simulink model "PVPAPERFULL"  (R2021b)
settings: Solver=VariableStepAuto  StartTime=0.0  StopTime=30.0  FixedStep=0.01  RelTol=1e-3
libraries: simulink x2, spsControlledCurrentSourceLib x1, spsControlledVoltageSourceLib x1, spsCurrentMeasurementLib x1, spsDiodeLib x1, spsVoltageMeasurementLib x1, spspowerguiLib x1
settings Model: Creator=shiuanlee  LastModifiedBy=Shiuan

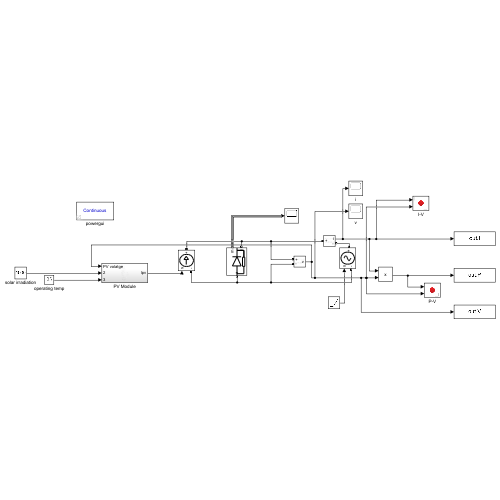
[thumbnail: Simulink's stored preview of the top-level diagram]
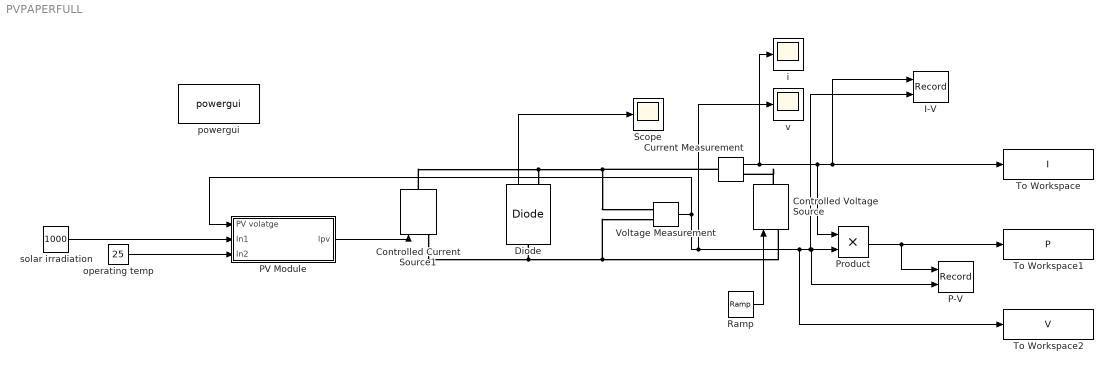
== system PVPAPERFULL ==
  Controlled Current Source1 : spsControlledCurrentSourceLib/Controlled Current Source  Initialize=on  Source_Type=AC  Amplitude=0  Phase=0  Frequency=0  Measurements=None
  Controlled Voltage Source : spsControlledVoltageSourceLib/Controlled Voltage Source  Initialize=on  Source_Type=AC  Amplitude=0  Phase=0  Frequency=0  Measurements=None
  Current Measurement : spsCurrentMeasurementLib/Current Measurement  PhasorSimulation=off  OutputType=Complex  PSBequivalent=0
  Diode : spsDiodeLib/Diode  Ron=0.001  Lon=0  Vf=0.8  IC=0  UseSnubber=0  Rs=500  Cs=250e-9  Measurements=on
  I-V : Record  FileSettingsInternal="{\"entries\":[{\"content\":{\"excelSettings\":{\"content\":{},\"type\":\"Streamout.ExcelSettings\"}},\"type\":\"Streamout.FileSettingStorage\",\"uuid\":\"36aaff03-e2d8-4f23-a0c3-637c8ac80c8f\"}],\"packageUris\":[\"http://schema.mathworks.com/mf0/streamout_blocks/R2020a\"],\"version\":\"1.0\"}"  Layout=[1 1]  SignalsInternal="{\"entries\":[{\"content\":{\"signals\":[{\"content\":{\"blockPath\":[\"PVPAPERFULL/I-V\"],\"channel\":[],\"dimensions\":[1],\"domain\":\"PVPAPERFULL/I-V\",\"lineColor\":\"#139fff\",\"plots\":[],\"port\":1,\"sid\":[\"\"],\"signalID\":2561,\"signalName\":\"Current Measurement\"},\"type\":\"RecordBlkView.Signal\",\"uuid\":\"db08aa17-c25b-43ab-bd0f-8571df5a55c5\"},{\"content\":{\"blockPath\":[\"PVPAPERFULL/I-V\"],\"channel\":[],\"dimensions\":[1],\"domain\":\"PVPAPERFULL/I-V\",\"lineColor\":\"#ff6929\",\"plots\":[],\"port\":2,\"sid\":[\"\"],\"signalID\":2565,\"signalName\":\"Voltage Measurement\"},\"type\":\"RecordBlkView.Signal\",\"uuid\":\"16e919e3-9877-4a22-964a-cc0445c3d14e\"}]},\"type\":\"RecordBlkView.InputSignals\",\"uuid\":\"2386edbf-e72d-401e-9176-175722332550\"}],\"packageUris\":[\"http://schema.mathworks.com/mf0/streamout_blocks/R2020a\"],\"version\":\"1.0\"}"  VisualizationBindings="{\"xyplotplugin\":{\"info\":[{\"series\":[],\"subplotID\":1}]}}"  CompatibilityTag=XY
  P-V : Record  FileSettingsInternal="{\"entries\":[{\"content\":{\"excelSettings\":{\"content\":{},\"type\":\"Streamout.ExcelSettings\"}},\"type\":\"Streamout.FileSettingStorage\",\"uuid\":\"6adaefe9-4cd2-429f-9127-09dd1fe31cef\"}],\"packageUris\":[\"http://schema.mathworks.com/mf0/streamout_blocks/R2020a\"],\"version\":\"1.0\"}"  Layout=[1 1]  SignalsInternal="{\"entries\":[{\"content\":{\"signals\":[{\"content\":{\"blockPath\":[\"PVPAPERFULL/P-V\"],\"channel\":[],\"dimensions\":[1],\"domain\":\"PVPAPERFULL/P-V\",\"lineColor\":\"#b746ff\",\"plots\":[],\"port\":1,\"sid\":[\"\"],\"signalID\":2569,\"signalName\":\"Product\"},\"type\":\"RecordBlkView.Signal\",\"uuid\":\"2bab4d67-adbc-4489-bddd-a9c0aabdc29e\"},{\"content\":{\"blockPath\":[\"PVPAPERFULL/P-V\"],\"channel\":[],\"dimensions\":[1],\"domain\":\"PVPAPERFULL/P-V\",\"lineColor\":\"#64d413\",\"plots\":[],\"port\":2,\"sid\":[\"\"],\"signalID\":2573,\"signalName\":\"Voltage Measurement\"},\"type\":\"RecordBlkView.Signal\",\"uuid\":\"ece211cf-a2a6-4dbd-807b-14eb8ce103a1\"}]},\"type\":\"RecordBlkView.InputSignals\",\"uuid\":\"0634f269-aaca-4857-9a94-01b50dbf8e93\"}],\"packageUris\":[\"http://schema.mathworks.com/mf0/streamout_blocks/R2020a\"],\"version\":\"1.0\"}"  VisualizationBindings="{\"xyplotplugin\":{\"info\":[{\"series\":[],\"subplotID\":1}]}}"  CompatibilityTag=XY
  PV Module : Subsystem
  Product : Product
  Ramp : simulink/Sources/Ramp  slope=1  start=0  InitialOutput=0
  Scope : Scope
  To Workspace : ToWorkspace  VariableName=I  SampleTime=-1
      settings: Save2DSignal=2-D array (concatenate along first dimension)
  To Workspace1 : ToWorkspace  VariableName=P  SampleTime=-1
      settings: Save2DSignal=2-D array (concatenate along first dimension)
  To Workspace2 : ToWorkspace  VariableName=V  SampleTime=-1
      settings: Save2DSignal=2-D array (concatenate along first dimension)
  Voltage Measurement : spsVoltageMeasurementLib/Voltage Measurement  PhasorSimulation=off  OutputType=Complex  PSBequivalent=0
  i : Scope
  operating temp : Constant  Value=25
  powergui : spspowerguiLib/powergui  Priority=1  SimulationMode=Continuous  SampleTime=50e-6  frequency=60  Iterations=50  frequencyindice=0  Pbase=100e6  ErrMax=1e-4  UnitsV=kV  UnitsW=MW  buscounter=0  FunctionMessages=off  echomessages=off  EnableUseOfTLC=off  CurrentSourceSwitches=off  DisableSnubberDevices=off  DisableRonSwitches=off  DisableVfSwitches=off  DisplayEquations=off  AutomaticDiscreteSolvers=off  SolverType=Tustin/Backward Euler (TBE)  Interpol=off  ExternalGateDelay=off  methode=off  Ts=100  x0status=blocks  SPID=on  SwTol=0  HookPort=off  NonlinearTolerance=1e-4  nMaxIteration=100  ContinueOnMaxIteration=off  RestoreLinks=warning  ResistiveCurrentMeasurement=off  Frange=[0:2:500]  Ylog=off  Xlog=on  ShowGrid=off  save=off  variable=ZData  structure=0  ZoomFFT=off  StartTime=0.0  cycles=1  DisplayStyle=1  fundamental=60  FreqAxis=off  MaxFrequency=1000  frequencyindicesteady=1  RmsSteady=1  display=off
  solar irradiation : Constant  Value=1000
  v : Scope
  wires:
  solar irradiation/1 -> PV Module/2(In1)
  operating temp/1 -> PV Module/3(In2)
  PV Module/1(lpv) -> Controlled Current Source1/1
  Diode/1 -> Scope/1
  Voltage Measurement/1 -> PV Module/1(PV volatge), I-V/2, P-V/2, Product/2, To Workspace2/1, v/1
  Ramp/1 -> Controlled Voltage Source/1
  Product/1 -> P-V/1, To Workspace1/1
  Current Measurement/1 -> i/1, Product/1, I-V/1, To Workspace/1
  connections:
  Controlled Current Source1/RConn1 -- Current Measurement/LConn1 -- Voltage Measurement/LConn1 -- Diode/RConn1
  Controlled Current Source1/LConn1 -- Voltage Measurement/LConn2 -- Controlled Voltage Source/LConn1 -- Diode/LConn1
  Controlled Voltage Source/RConn1 -- Current Measurement/RConn1

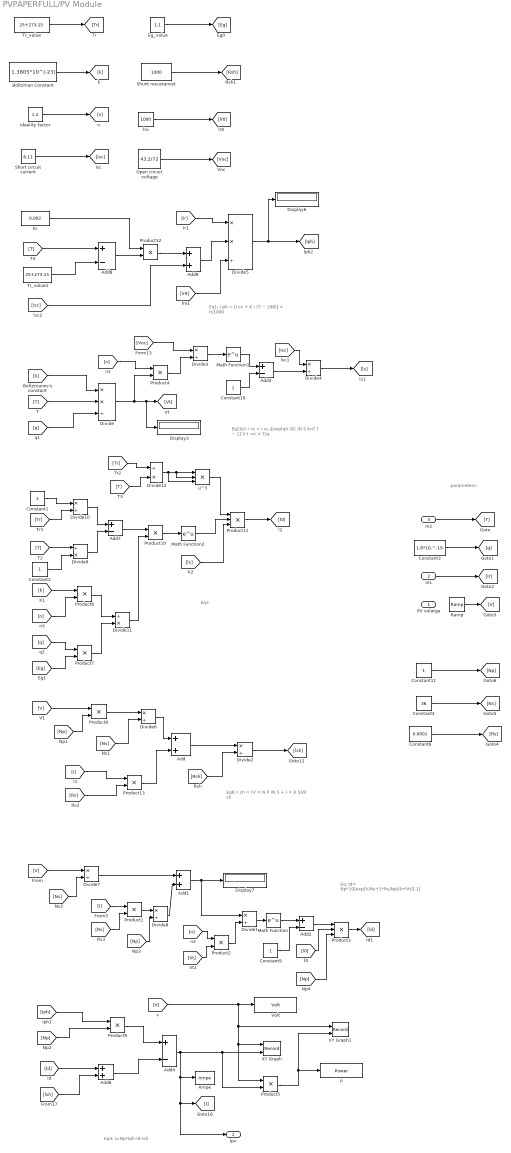
== system PVPAPERFULL/PV Module ==
  note: Eq4:
      | I=Np*Iph-Id-Ish
  note: Eq6:
      | I sh = (V × N P /N S + I × R S)/R sh
  note: Eq1:
      | I ph = [I sc + K i (T − 298)] × Ir/1000
  note: Eq:
      | Id= Np*10[exp[V/Ns+1*Rs/Np)/(n*Vt)]-1]
  note: Eq2&5:
      | I rs = I sc /[exp(qV OC /N S knT ) − 1]
      | V t =k × T/q
  note: parameters:
  note: Eq3
  PV volatge : Inport
  In1 : Inport  Port=2
  In2 : Inport  Port=3
  Add{,1,6,9} (4 alike) : Sum
  Add{2..4,7..8} (5 alike) : Sum  Inputs=+-
  Ampe : ToWorkspace  VariableName=Ampe  SaveFormat=Timeseries  SampleTime=-1
  Boltzman Constant : Constant  Value=1.3805*10^(-23)
  Constant{1..2,9..11} (5 alike) : Constant
  Constant3 : Constant  Value=1.6*10.^-19
  Constant4 : Constant  Value=36
  Constant6 : Constant  Value=0.0001
  Display3 : Display
  Display6 : Display
  Display7 : Display
  Divide : Product  Inputs=**/
  Divide{1..4,6..8,10} (8 alike) : Product  Inputs=*/
  Divide11 : Product  Inputs=/*
  Divide12 : Product  Inputs=/*
  Divide5 : Product  Inputs=**/
  Divide9 : Product  Inputs=/*
  Eg_value : Constant  Value=1.1
  Ideality factor : Constant  Value=1.2
  Ki : Constant  Value=0.002
  Math Function : Math  SaturateOnIntegerOverflow=on
  Math Function1 : Math  SaturateOnIntegerOverflow=on
  Math Function2 : Math  SaturateOnIntegerOverflow=on
  Open circuit voltage : Constant  Value=43.2/72
  P : ToWorkspace  VariableName=Power  SaveFormat=Timeseries  SampleTime=-1
  Product{1..2,4..10,12..13} (11 alike) : Product
  Product11 : Product  Inputs=3
  Product3 : Product  Inputs=3
  Ramp : simulink/Sources/Ramp  slope=1  start=0  InitialOutput=0
  Short circuit current : Constant  Value=6.11
  Shunt resustancet : Constant  Value=1000
  Tr_value : Constant  Value=25+273.15
  Tr_value1 : Constant  Value=25+273.15
  Volt : ToWorkspace  VariableName=Volt  SaveFormat=Timeseries  SampleTime=-1
  XY Graph : Record  FileSettingsInternal="{\"entries\":[{\"content\":{\"excelSettings\":{\"content\":{},\"type\":\"Streamout.ExcelSettings\"}},\"type\":\"Streamout.FileSettingStorage\",\"uuid\":\"ab1ddb20-419f-491b-9c58-684249219fa2\"}],\"packageUris\":[\"http://schema.mathworks.com/mf0/streamout_blocks/R2020a\"],\"version\":\"1.0\"}"  Layout=[1 1]  SignalsInternal="{\"entries\":[{\"content\":{\"signals\":[{\"content\":{\"blockPath\":[\"PVPAPERFULL/PV Module/XY Graph\"],\"channel\":[],\"dimensions\":[1],\"domain\":\"PVPAPERFULL/PV Module/XY Graph\",\"lineColor\":\"#ff13a6\",\"plots\":[],\"port\":1,\"sid\":[\"\"],\"signalID\":2577,\"signalName\":\"v\"},\"type\":\"RecordBlkView.Signal\",\"uuid\":\"b3b8c47f-d49e-40f3-9268-4f0746602f4a\"},{\"content\":{\"blockPath\":[\"PVPAPERFULL/PV Module/XY Graph\"],\"channel\":[],\"dimensions\":[1],\"domain\":\"PVPAPERFULL/PV Module/XY Graph\",\"lineColor\":\"#fe330a\",\"plots\":[],\"port\":2,\"sid\":[\"\"],\"signalID\":2581,\"signalName\":\"Add4\"},\"type\":\"RecordBlkView.Signal\",\"uuid\":\"6a1236be-1971-4489-abe7-72c75e1e56dd\"}]},\"type\":\"RecordBlkView.InputSignals\",\"uuid\":\"4581ca48-da48-410f-b8a3-f7acb8399d5c\"}],\"packageUris\":[\"http://schema.mathworks.com/mf0/streamout_blocks/R2020a\"],\"version\":\"1.0\"}"  CompatibilityTag=XY
  XY Graph1 : Record  FileSettingsInternal="{\"entries\":[{\"content\":{\"excelSettings\":{\"content\":{},\"type\":\"Streamout.ExcelSettings\"}},\"type\":\"Streamout.FileSettingStorage\",\"uuid\":\"4447556a-2442-499e-ba43-95e3cd0e45cb\"}],\"packageUris\":[\"http://schema.mathworks.com/mf0/streamout_blocks/R2020a\"],\"version\":\"1.0\"}"  Layout=[1 1]  SignalsInternal="{\"entries\":[{\"content\":{\"signals\":[{\"content\":{\"blockPath\":[\"PVPAPERFULL/PV Module/XY Graph1\"],\"channel\":[],\"dimensions\":[1],\"domain\":\"PVPAPERFULL/PV Module/XY Graph1\",\"lineColor\":\"#22b573\",\"plots\":[],\"port\":1,\"sid\":[\"\"],\"signalID\":2585,\"signalName\":\"v\"},\"type\":\"RecordBlkView.Signal\",\"uuid\":\"bc056c73-eab7-4f39-8a85-5b50627b3442\"},{\"content\":{\"blockPath\":[\"PVPAPERFULL/PV Module/XY Graph1\"],\"channel\":[],\"dimensions\":[1],\"domain\":\"PVPAPERFULL/PV Module/XY Graph1\",\"lineColor\":\"#0072bd\",\"plots\":[],\"port\":2,\"sid\":[\"\"],\"signalID\":2589,\"signalName\":\"Product5\"},\"type\":\"RecordBlkView.Signal\",\"uuid\":\"cc3d43ba-43ff-43cb-8563-964e4b65ad12\"}]},\"type\":\"RecordBlkView.InputSignals\",\"uuid\":\"8793bc40-c625-4f15-adda-cfc5e14292cf\"}],\"packageUris\":[\"http://schema.mathworks.com/mf0/streamout_blocks/R2020a\"],\"version\":\"1.0\"}"  VisualizationBindings="{\"xyplotplugin\":{\"info\":[{\"series\":[],\"subplotID\":1}]}}"  CompatibilityTag=XY
  lro : Constant  Value=1000
  u^3 : Product  Inputs=3
  lpv : Outport
  wires:
  [Np] -> Product9/2
  [ld] -> Add6/1
  Divide1/1 -> Math Function/1
  Product3/1 -> [ld]
  Constant9/1 -> Add2/2
  Boltzman Constant/1 -> [k]
  Math Function1/1 -> Add3/1
  [Tr] -> Divide12/1
  Divide9/1 -> Add7/2
  Product5/1 -> XY Graph1/2, P/1
  [Np] -> Divide8/2
  Tr_value1/1 -> Add8/2
  Constant11/1 -> [Np]
  [lsh] -> Add6/2
  [V] -> Volt/1, XY Graph1/1, Product5/1, XY Graph/1
  Tr_value/1 -> [Tr]
  Ki/1 -> Product12/1
  Product12/1 -> Add9/1
  [n] -> Product6/2
  [Vt] -> Product2/2
  Product7/1 -> Divide11/2
  Math Function2/1 -> Product11/2
  Constant3/1 -> [q]
  Constant4/1 -> [Ns]
  Product10/1 -> Math Function2/1
  [Ns] -> Divide7/2
  Math Function/1 -> Add2/1
  [lr0] -> Divide5/3
  [Np] -> Product3/3
  [Iph] -> Product9/1
  [ls] -> Product11/3
  Constant6/1 -> [Rs]
  Constant2/1 -> Divide9/2
  Divide/1 -> Display3/1, [Vt], Product4/2
  Constant10/1 -> Add3/2
  Divide2/1 -> [lsh]
  Add2/1 -> Product3/1
  [T] -> Divide12/2
  Product2/1 -> Divide1/2
  [I] -> Product1/1
  Product1/1 -> Divide8/1
  [l0] -> Product3/2
  Divide8/1 -> Add1/2
  [n] -> Product2/1
  Product13/1 -> Add/2
  Add1/1 -> Divide1/1, Display7/1
  Open circuit voltage/1 -> [Voc]
  [V] -> Divide7/1
  [Ns] -> Divide6/2
  [Rs] -> Product1/2
  [k] -> Product6/1
  [Isc] -> Add9/2
  Divide3/1 -> Math Function1/1
  [T] -> Add8/1
  Ideality factor/1 -> [n]
  Product8/1 -> Divide6/1
  [Tr] -> Divide10/2
  Add7/1 -> Product10/1
  [V] -> Product8/1
  [q] -> Product7/1
  Divide11/1 -> Product10/2
  Divide10/1 -> Add7/1
  [Np] -> Product8/2
  [T] -> Divide9/1
  u^3/1 -> Product11/1
  Product6/1 -> Divide11/1
  Constant1/1 -> Divide10/1
  Product11/1 -> [l0]
  [Eg] -> Product7/2
  [Isc] -> Divide4/1
  [k] -> Divide/1
  Divide6/1 -> Add/1
  Add8/1 -> Product12/2
  [Rs] -> Product13/2
  Product4/1 -> Divide3/2
  lro/1 -> [lr0]
  [Rsh] -> Divide2/2
  Divide12/1 -> u^3/3, u^3/2, u^3/1
  [n] -> Product4/1
  [q] -> Divide/3
  [I] -> Product13/1
  Add/1 -> Divide2/1
  [T] -> Divide/2
  Add9/1 -> Divide5/2
  Divide7/1 -> Add1/1
  Eg_value/1 -> [Eg]
  Divide5/1 -> Display6/1, [Iph]
  Divide4/1 -> [ls]
  Add3/1 -> Divide4/2
  Shunt resustancet/1 -> [Rsh]
  [Voc] -> Divide3/1
  Short circuit current/1 -> [Isc]
  [Ir] -> Divide5/1
  Add4/1 -> XY Graph/2, Product5/2, [I], lpv/1, Ampe/1
  In2/1 -> [T]
  In1/1 -> [Ir]
  Product9/1 -> Add4/1
  Add6/1 -> Add4/2
  Ramp/1 -> [V]
